simulink model "rtMotomanVR"  (R2019b)
settings: Solver=FixedStepDiscrete  StartTime=0.0  StopTime=8  FixedStep=dT  RelTol=1e-3  EnableMultiTasking=on
values from neighbouring files (symbols this model uses):
  dT = 1/500    (= 0.002)    [initVR.m]    (also in trajectory.m = 0.00025)
libraries: xpcutilitieslib x2, dspnetwork x2, simulink x1
Description:
  | Real-Time Van der Pol Simulation
  | 
  | This demonstration shows a real-time version of the Simulink Van der Pol
  | simulation demo. This model does not need any external signals, so it does
  | not need any data acquisition hardware or driver. This makes the model ideal
  | for first experiments with Real-Time Windows Target, without need to
  | worry about proper I/O hardware configuration.
  | 
  | How to run this demo:
  | 
  |   1. Build the model using Tools -> Real-Time Workshop -> Build Model.
  |   2. Connect to the real-time code using Simulation -> Connect to target.
  |   3. Start the real-time execution using Simulation -> Start real-time code.
settings Model: EnablePacing=on  Creator=Houska  LastModifiedBy=Sebastjan
settings DataIOCC: LimitDataPoints=on  SaveFormat=Array  SignalLoggingSaveFormat=ModelDataLogs  SaveOutput=off  SaveTime=off  ReturnWorkspaceOutputs=off  SignalLoggingName=logsOut
settings OptimizationCC: ExpressionDepthLimit=2147483647  InitFltsAndDblsToZero=on  LifeSpan=inf
settings DebuggingCC: SaveWithParameterizedLinksMsg=none  UnderspecifiedInitializationDetection=Classic  MergeDetectMultiDrivingBlocksExec=none  SignalResolutionControl=TryResolveAllWithWarning  MultiTaskDSMMsg=warning  MultiTaskCondExecSysMsg=none  FcnCallInpInsideContextMsg=warning  StateNameClashWarn=warning  SFUnexpectedBacktrackingDiag=warning  SFNoUnconditionalDefaultTransitionDiag=warning  SFExecutionAtInitializationDiag=none  ArithmeticOperatorsInVariantConditions=warning
settings HardwareCC: ProdBitPerPointer=32  ProdBitPerSizeT=32  ProdBitPerPtrDiffT=32  ProdLargestAtomicFloat=None  ProdWordSize=32  ProdHWDeviceType=32-bit Real-Time Windows Target
settings ModelReferenceCC: PropagateSignalLabelsOutOfModel=off
settings SFSimCC: SimUseLocalCustomCode=off  SimParseCustomCode=off  CustomCodeUndefinedFunction=UseInterfaceOnly
settings RTWCC: Description=Real-Time Windows Target  SystemTargetFile=rtwin.tlc  TemplateMakefile=rtwin.tmf  RTWUseLocalCustomCode=off
settings CodeAppCC: StateflowObjectComments=on
settings TargetCC: TargetFcnLib=ansi_tfl_tmw.mat  ModelReferenceCompliant=off  CompOptLevelCompliant=off  PreserveStateflowLocalDataDimensions=off
settings ConfigComp: CovMetricSettings=dw  CovHtmlReporting=on  CovSaveCumulativeToWorkspaceVar=on  CovSaveSingleToWorkspaceVar=on  CovExternalEMLEnable=off

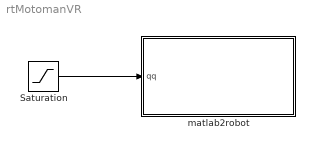
== system rtMotomanVR ==
  Saturation : Saturate  UpperLimit=([94.5, 75, 45, 160, 120 180]-5)*pi/180  LowerLimit=([-94.5, -40, -75, -160, -120, -180]+5)*pi/180
  matlab2robot : Subsystem  mask{selUDP=Simulacija, slrt_ip='192.168.65.250', slrt_port=55555, sampleTime=dT}
      mask prompts: selUDP "Izvajanje programa:"; slrt_ip "Simulink Real Time IP:"; slrt_port "Simulink Real Time Port:"; sampleTime "Vzorcni cas:"
      mask init:
      | switch selUDP
      |     case 1
      |         enSim = 1;
      |         enRob = 0;
      |     case 2
      |         enSim = 0;
      |         enRob = 1;
      |     otherwise
      |         enSim = 0;
      |         enRob = 0;
      | end
      mask TypeOptions selUDP: Simulacija | Robot
  wires:
  Saturation/1 -> matlab2robot/1(qq)

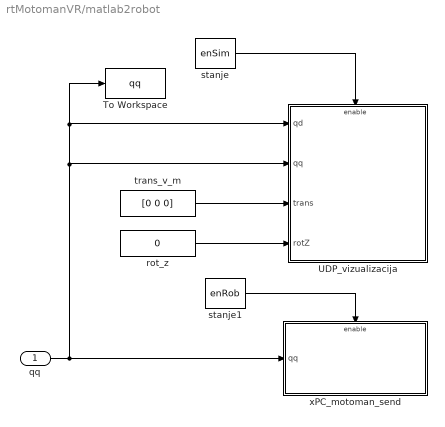
== system rtMotomanVR/matlab2robot ==
  qq : Inport
  To Workspace : ToWorkspace  VariableName=qq  SampleTime=-1
  UDP_vizualizacija : Subsystem
  rot_z : Constant  Value=0
  stanje : Constant  Value=enSim  SampleTime=dT
  stanje1 : Constant  Value=enRob  SampleTime=dT
  trans_v_m : Constant  Value=[0 0 0]
  xPC_motoman_send : Subsystem  mask{IDSeje=rand(1), GetReady=1, slrt_ip1=slrt_ip, slrt_port1=slrt_port}
      mask prompts: IDSeje "IDSeje Function"; GetReady "GetReady Function"; slrt_ip1 "xPC Target IP"; slrt_port1 "xPC Target port"
      mask init:
      | %set_param([gcb,'/Send'],'remoteURL',slrt_ip1);
      | %set_param([gcb,'/Send'],'remotePort',num2str(slrt_port1));
      mask Callback slrt_port1: % set_param([gcb,'/Send'],'ipPort',slrt_port)
  wires:
  stanje/1 -> UDP_vizualizacija/Enable
  rot_z/1 -> UDP_vizualizacija/4(rotZ)
  trans_v_m/1 -> UDP_vizualizacija/3(trans)
  qq/1 -> To Workspace/1, UDP_vizualizacija/1(qd), UDP_vizualizacija/2(qq), xPC_motoman_send/1(qq)
  stanje1/1 -> xPC_motoman_send/Enable

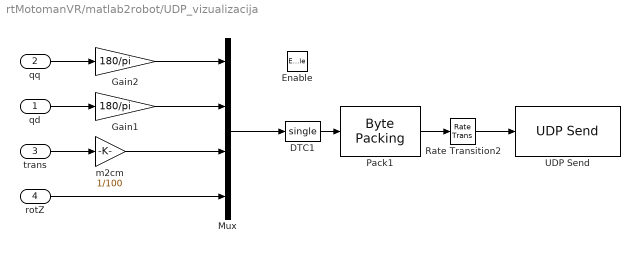
== system rtMotomanVR/matlab2robot/UDP_vizualizacija ==
  qd : Inport
  qq : Inport  Port=2
  trans : Inport  Port=3
  rotZ : Inport  Port=4
  Enable : EnablePort  StatesWhenEnabling=reset
  DTC1 : DataTypeConversion  OutDataTypeStr=single
  Gain1 : Gain  Gain=180/pi
  Gain2 : Gain  Gain=180/pi
  Mux : Mux
  Pack1 : xpcutilitieslib/Byte Packing   MaskPackedDataType=uint8  MaskUnpackedDataTypes={'single'}  MaskAlignment=1
  Rate Transition2 : RateTransition
  UDP Send : dspnetwork/UDP Send  remoteURL='127.0.0.1'  remotePort=25300  localURL='0.0.0.0'  localPortSource=Automatically determine  localPort=-1  sampletime=-1  blockPlatform=[]  separateLengthPort=0
      settings: SourceProductName=Simulink
  m2cm : Gain  Gain=1/100
  wires:
  trans/1 -> m2cm/1
  Mux/1 -> DTC1/1
  m2cm/1 -> Mux/3
  rotZ/1 -> Mux/4
  qq/1 -> Gain2/1
  qd/1 -> Gain1/1
  Gain2/1 -> Mux/1
  Gain1/1 -> Mux/2
  Pack1/1 -> Rate Transition2/1
  Rate Transition2/1 -> UDP Send/1
  DTC1/1 -> Pack1/1

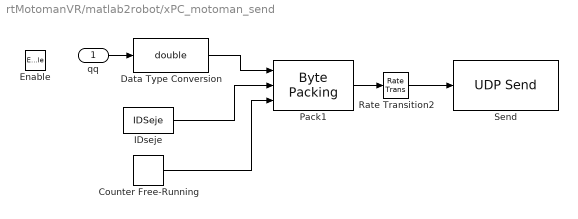
== system rtMotomanVR/matlab2robot/xPC_motoman_send ==
  qq : Inport
  Enable : EnablePort  StatesWhenEnabling=reset
  Counter Free-Running : simulink/Sources/Counter Free-Running  NumBits=16  tsamp=-1
  Data Type Conversion : DataTypeConversion  OutDataTypeStr=double  SampleTime=dT
  IDseje : Constant  Value=IDSeje  SampleTime=dT
  Pack1 : xpcutilitieslib/Byte Packing   MaskPackedDataType=uint8  MaskUnpackedDataTypes={'double','double','uint16'}  MaskAlignment=1
  Rate Transition2 : RateTransition
  Send : dspnetwork/UDP Send  remoteURL='192.168.65.250'  remotePort=55555  localURL='0.0.0.0'  localPortSource=Automatically determine  localPort=-1  sampletime=-1  blockPlatform=[]  separateLengthPort=0
      settings: SourceProductName=Simulink
  wires:
  qq/1 -> Data Type Conversion/1
  IDseje/1 -> Pack1/2
  Data Type Conversion/1 -> Pack1/1
  Counter Free-Running/1 -> Pack1/3
  Pack1/1 -> Rate Transition2/1
  Rate Transition2/1 -> Send/1
